simulink model "TF_Check"  (R2018a)
settings: Solver=ode23t  StartTime=0.0  StopTime=0.6  RelTol=1e-3  AbsTol=1e-3  EnableMultiTasking=on
values from neighbouring files (symbols this model uses):
  C1 = 200e-6    (= 0.0002)    [ChopperRmsSIm.m]    (also in test_TFCheck.m)
  C1_ESL = 1e-9    (= 1e-09)    [ChopperRmsSIm.m]    (also in test_TFCheck.m)
  C1_ESR = 1e-3    (= 0.001)    [ChopperRmsSIm.m]    (also in test_TFCheck.m)
  C2 = 1000e-6    (= 0.001)    [ChopperRmsSIm.m]    (also in test_TFCheck.m)
  C2_ESL = 1e-9    (= 1e-09)    [ChopperRmsSIm.m]    (also in test_TFCheck.m)
  C2_ESR = 1e-3    (= 0.001)    [ChopperRmsSIm.m]    (also in test_TFCheck.m)
  C_smooth = 400e-6    (= 0.0004)    [ChopperRmsSIm.m]    (also in test_TFCheck.m)
  current_source = 5.0    (= 5)    [ChopperRmsSIm.m]    (also in test_TFCheck.m)
  L1 = 1e-6    (= 1e-06)    [ChopperRmsSIm.m]    (also in test_TFCheck.m)
  L1_R = 1e-3    (= 0.001)    [ChopperRmsSIm.m]    (also in test_TFCheck.m)
  L2 = 1e-6    (= 1e-06)    [ChopperRmsSIm.m]    (also in test_TFCheck.m)
  L2_R = 1e-3    (= 0.001)    [ChopperRmsSIm.m]    (also in test_TFCheck.m)
  L_cable = 10e-6    (= 1e-05)    [ChopperRmsSIm.m]    (also in test_TFCheck.m)
  R_cable = 12e-3    (= 0.012)    [ChopperRmsSIm.m]    (also in test_TFCheck.m)
  sample_time = 1e-6    (= 1e-06)    [ChopperRmsSIm.m]    (also in test_TFCheck.m)
  Vdc = 50    [ChopperRmsSIm.m]    (also in test_TFCheck.m)
undefined symbols (not defined in the file or in its folder): aaa
libraries: powerlib x18, simulink x1
settings Model: Creator=snow_  LastModifiedBy=snow_
settings SolverCC: AutoScaleAbsTol=off
settings DataIOCC: LimitDataPoints=on  MaxDataPoints=10000
settings OptimizationCC: LifeSpan=inf
settings DebuggingCC: AllowSymbolicDim=off  SFUnexpectedBacktrackingDiag=warning  SFNoUnconditionalDefaultTransitionDiag=warning  SFExecutionAtInitializationDiag=none
settings CodeAppCC: StateflowObjectComments=on
settings GRTTargetCC: TargetLangStandard=C89/C90 (ANSI)  GeneratePreprocessorConditionals=Disable all
settings ConfigComp: CovMetricSettings=dw  CovHtmlReporting=on  CovSaveCumulativeToWorkspaceVar=on  CovSaveSingleToWorkspaceVar=on  CovExternalEMLEnable=off  CovSFcnEnable=off
settings SimscapeCC: SimscapeLogType=all  SimscapeLogDataHistory=10000

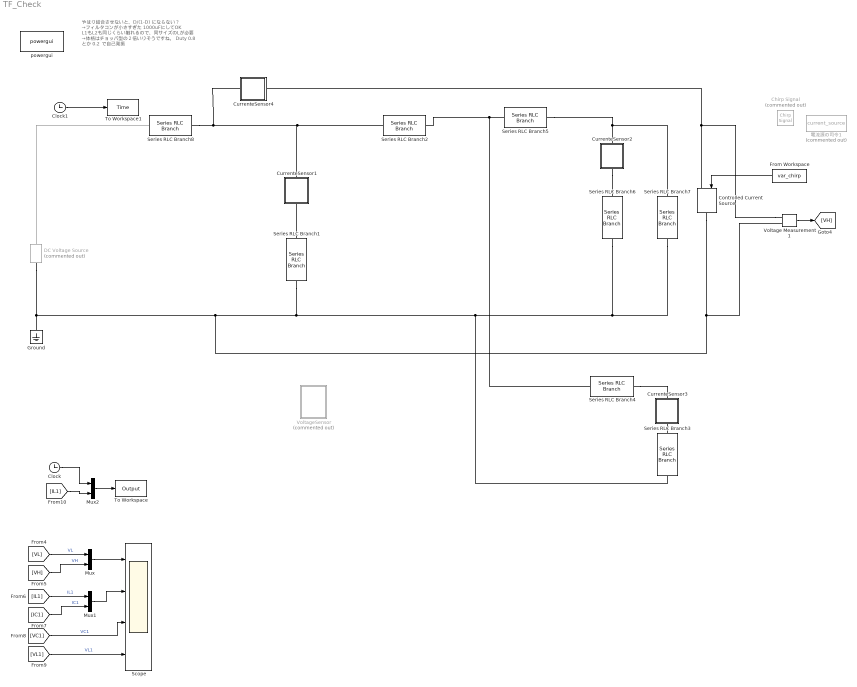
== system TF_Check ==
  note: やはり結合させないと、D/(1-D)　にならない？
      | →フィルタコンが小さすぎた　1000uFにしてOK
      |
      | L1もL2も同じくらい触れるので、同サイズのLが必要
      | →体格はチョッパ型の２倍いりそうですね。
      |
      | Duty 0.8 とか　0.2 で自己発振
  Chirp Signal : simulink/Sources/Chirp Signal  Commented=on  f1=1  T=0.3  f2=50000
  Clock : Clock
  Clock1 : Clock
  Controlled Current Source : powerlib/Electrical Sources/Controlled Current Source  Initialize=on  Source_Type=AC  Amplitude=0  Phase=0  Frequency=0  Measurements=None
  CurrenteSensor1 : Subsystem
  CurrenteSensor2 : Subsystem
  CurrenteSensor3 : Subsystem
  CurrenteSensor4 : Subsystem
  DC Voltage Source : powerlib/Electrical Sources/DC Voltage Source  Commented=on  Amplitude=Vdc  Measurements=None
      settings: AttributesFormatString=DC = %<Amplitude> V
  From Workspace : FromWorkspace  VariableName=var_chirp  SampleTime=sample_time
  Ground : powerlib/Elements/Ground  LConnTagsString=a
  Mux : Mux  Inputs=2
  Mux1 : Mux  Inputs=2
  Mux2 : Mux  Inputs=2
  Scope : Scope  NumInputPorts=4
  Series RLC Branch1 : powerlib/Elements/Series RLC Branch  LConnTagsString=__new0  RConnTagsString=__new0  BranchType=C  Resistance=24e-3  Inductance=1000e-6  SetiL0=off  InitialCurrent=0  Capacitance=C_smooth  Setx0=on  InitialVoltage=Vdc  Measurements=None
      settings: AttributesFormatString="C= %<Capacitance>  F"
  Series RLC Branch2 : powerlib/Elements/Series RLC Branch  LConnTagsString=__new0  RConnTagsString=__new0  BranchType=RL  Resistance=R_cable  Inductance=L_cable  SetiL0=off  InitialCurrent=0  Capacitance=1e-6  Setx0=off  InitialVoltage=0  Measurements=None
      settings: AttributesFormatString=|
      | L=%<Inductance> H
      | R=%<Resistance> Ohm
  Series RLC Branch3 : powerlib/Elements/Series RLC Branch  LConnTagsString=__new0  RConnTagsString=__new0  BranchType=RLC  Resistance=C1_ESR  Inductance=C1_ESL  SetiL0=off  InitialCurrent=0  Capacitance=C1  Setx0=off  InitialVoltage=0  Measurements=None
      settings: AttributesFormatString=|
      | L=%<Inductance> H
      | R=%<Resistance> Ohm
  Series RLC Branch4 : powerlib/Elements/Series RLC Branch  LConnTagsString=__new0  RConnTagsString=__new0  BranchType=RL  Resistance=L1_R  Inductance=L1  SetiL0=off  InitialCurrent=0  Capacitance=1e-6  Setx0=off  InitialVoltage=0  Measurements=None
      settings: AttributesFormatString=|
      | L=%<Inductance> H
      | R=%<Resistance> Ohm
  Series RLC Branch5 : powerlib/Elements/Series RLC Branch  LConnTagsString=__new0  RConnTagsString=__new0  BranchType=RL  Resistance=L2_R  Inductance=L2  SetiL0=off  InitialCurrent=0  Capacitance=1e-6  Setx0=off  InitialVoltage=0  Measurements=None
      settings: AttributesFormatString=|
      | L=%<Inductance> H
      | R=%<Resistance> Ohm
  Series RLC Branch6 : powerlib/Elements/Series RLC Branch  LConnTagsString=__new0  RConnTagsString=__new0  BranchType=RLC  Resistance=C2_ESR  Inductance=C2_ESL  SetiL0=off  InitialCurrent=0  Capacitance=C2  Setx0=off  InitialVoltage=0  Measurements=None
      settings: AttributesFormatString=|
      | L=%<Inductance> H
      | R=%<Resistance> Ohm
  Series RLC Branch7 : powerlib/Elements/Series RLC Branch  LConnTagsString=__new0  RConnTagsString=__new0  BranchType=R  Resistance=100e3  Inductance=C2_ESL  SetiL0=off  InitialCurrent=0  Capacitance=C2  Setx0=off  InitialVoltage=0  Measurements=None
      settings: AttributesFormatString=R=%<Resistance> Ohm
  Series RLC Branch8 : powerlib/Elements/Series RLC Branch  LConnTagsString=__new0  RConnTagsString=__new0  BranchType=R  Resistance=1e-6  Inductance=C2_ESL  SetiL0=off  InitialCurrent=0  Capacitance=C2  Setx0=off  InitialVoltage=0  Measurements=None
      settings: AttributesFormatString=R=%<Resistance> Ohm
  To Workspace : ToWorkspace  VariableName=Output  SampleTime=sample_time
  To Workspace1 : ToWorkspace  VariableName=Time  SampleTime=sample_time
  Voltage Measurement1 : powerlib/Measurements/Voltage Measurement  PhasorSimulation=off  OutputType=Complex  PSBequivalent=0
  VoltageSensor : Subsystem  Commented=on  mask{Val=aaa, SampleTime=1e-6}
      mask prompts: Val "VariableName"
      mask Display: disp("Voltage \n Sensor")
  powergui : powerlib/powergui  Priority=1  SimulationMode=Continuous  SampleTime=50e-6  frequency=60  Iterations=50  frequencyindice=0  Pbase=100e6  ErrMax=1e-4  UnitsV=kV  UnitsW=MW  buscounter=0  FunctionMessages=off  echomessages=off  EnableUseOfTLC=off  CurrentSourceSwitches=off  DisableSnubberDevices=off  DisableRonSwitches=off  DisableVfSwitches=off  DisplayEquations=off  SolverType=Tustin/Backward Euler (TBE)  Interpol=off  ExternalGateDelay=off  methode=off  Ts=100  x0status=blocks  SPID=on  SwTol=0  HookPort=off  RestoreLinks=warning  ResistiveCurrentMeasurement=off  Frange=[0:2:500]  Ylog=off  Xlog=on  ShowGrid=off  save=off  variable=ZData  structure=0  ZoomFFT=off  StartTime=0.0  cycles=1  DisplayStyle=1  fundamental=60  FreqAxis=off  MaxFrequency=1000  frequencyindicesteady=1  RmsSteady=1  display=off
  電流源の司令1 : Constant  Commented=on  Value=current_source
  wires:
  Mux/1 -> Scope/1
  Voltage Measurement1/1 -> [VH]
  [VL] -> Mux/1  "VL"
  [VH] -> Mux/2  "VH"
  [IL1] -> Mux1/1  "IL1"
  [IC1] -> Mux1/2  "IC1"
  Mux1/1 -> Scope/2
  [VC1] -> Scope/3  "VC1"
  [VL1] -> Scope/4  "VL1"
  [IL1] -> Mux2/2
  Clock/1 -> Mux2/1
  Mux2/1 -> To Workspace/1
  From Workspace/1 -> Controlled Current Source/1
  Clock1/1 -> To Workspace1/1
  connections:
  Series RLC Branch4/LConn1 -- Series RLC Branch5/LConn1 -- Series RLC Branch2/RConn1
  Controlled Current Source/RConn1 -- Series RLC Branch7/RConn1 -- Series RLC Branch6/RConn1 -- Series RLC Branch3/RConn1 -- Series RLC Branch1/RConn1 -- Ground/LConn1 -- DC Voltage Source/LConn1 -- Voltage Measurement1/LConn2
  DC Voltage Source/RConn1 -- Series RLC Branch8/LConn1
  CurrenteSensor3/RConn1 -- Series RLC Branch3/LConn1
  CurrenteSensor2/RConn1 -- Series RLC Branch6/LConn1
  Series RLC Branch8/RConn1 -- CurrenteSensor4/LConn1 -- Series RLC Branch2/LConn1 -- CurrenteSensor1/LConn1
  Series RLC Branch1/LConn1 -- CurrenteSensor1/RConn1
  Series RLC Branch7/LConn1 -- Series RLC Branch5/RConn1 -- CurrenteSensor2/LConn1
  Series RLC Branch4/RConn1 -- CurrenteSensor3/LConn1
  Voltage Measurement1/LConn1 -- Controlled Current Source/LConn1 -- CurrenteSensor4/RConn1

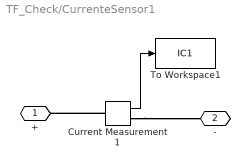
== system TF_Check/CurrenteSensor1 ==
  Current Measurement1 : powerlib/Measurements/Current Measurement  PhasorSimulation=off  OutputType=Complex  PSBequivalent=0
  To Workspace1 : ToWorkspace  VariableName=IC1  SampleTime=sample_time
  + : PMIOPort  Side=Left
  - : PMIOPort  Port=2  Side=Right
  wires:
  Current Measurement1/1 -> To Workspace1/1
  connections:
  Current Measurement1/LConn1 -- +/RConn1
  Current Measurement1/RConn1 -- -/RConn1

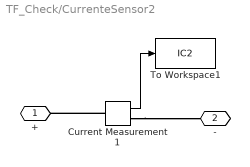
== system TF_Check/CurrenteSensor2 ==
  Current Measurement1 : powerlib/Measurements/Current Measurement  PhasorSimulation=off  OutputType=Complex  PSBequivalent=0
  To Workspace1 : ToWorkspace  VariableName=IC2  SampleTime=sample_time
  + : PMIOPort  Side=Left
  - : PMIOPort  Port=2  Side=Right
  wires:
  Current Measurement1/1 -> To Workspace1/1
  connections:
  Current Measurement1/LConn1 -- +/RConn1
  Current Measurement1/RConn1 -- -/RConn1

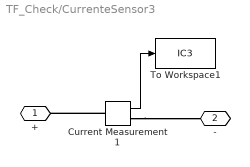
== system TF_Check/CurrenteSensor3 ==
  Current Measurement1 : powerlib/Measurements/Current Measurement  PhasorSimulation=off  OutputType=Complex  PSBequivalent=0
  To Workspace1 : ToWorkspace  VariableName=IC3  SampleTime=sample_time
  + : PMIOPort  Side=Left
  - : PMIOPort  Port=2  Side=Right
  wires:
  Current Measurement1/1 -> To Workspace1/1
  connections:
  Current Measurement1/LConn1 -- +/RConn1
  Current Measurement1/RConn1 -- -/RConn1

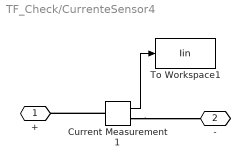
== system TF_Check/CurrenteSensor4 ==
  Current Measurement1 : powerlib/Measurements/Current Measurement  PhasorSimulation=off  OutputType=Complex  PSBequivalent=0
  To Workspace1 : ToWorkspace  VariableName=Iin  SampleTime=sample_time
  + : PMIOPort  Side=Left
  - : PMIOPort  Port=2  Side=Right
  wires:
  Current Measurement1/1 -> To Workspace1/1
  connections:
  Current Measurement1/LConn1 -- +/RConn1
  Current Measurement1/RConn1 -- -/RConn1

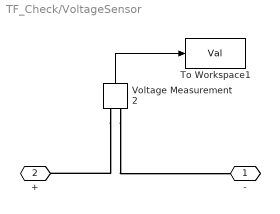
== system TF_Check/VoltageSensor ==
  To Workspace1 : ToWorkspace  VariableName=Val  SampleTime=SampleTime
  Voltage Measurement2 : powerlib/Measurements/Voltage Measurement  PhasorSimulation=off  OutputType=Complex  PSBequivalent=0
  - : PMIOPort  Side=Left
  + : PMIOPort  Port=2  Side=Left
  wires:
  Voltage Measurement2/1 -> To Workspace1/1
  connections:
  Voltage Measurement2/LConn1 -- +/RConn1
  Voltage Measurement2/LConn2 -- -/RConn1
